simulink model "bmsfinal"  (R2026a)
settings: Solver=VariableStepAuto  StopTime=1000.0
libraries: fl_lib x3, nesl_utility x3, ee_lib x1, batteryecm_lib x1
settings Model: LastModifiedBy=amrut

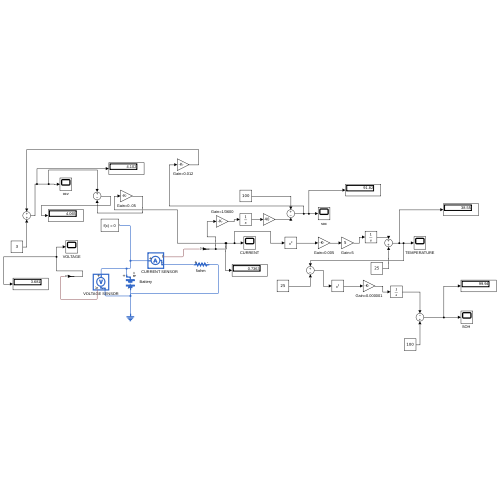
[thumbnail: Simulink's stored preview of the top-level diagram]
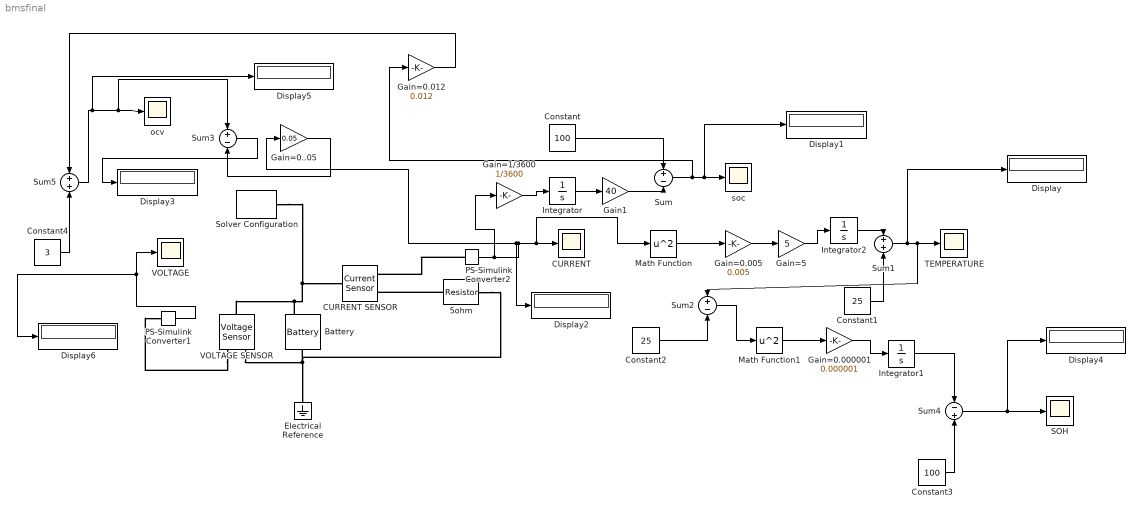
== system bmsfinal ==
  "          CURRENT SENSOR   " : fl_lib/Electrical/Electrical Sensors/Current Sensor
  5ohm : ee_lib/Passive/Resistor  R=5 Ohm  enable_R_tol=ee.enum.toleranceApplication.none  R_tol=5  tol_distribution=ee.enum.toleranceDistribution.uniform  nSigma=4  enable_operating_limits=ee.enum.enable.no  operating_limit_action=ee.enum.passive.reportOpLim.warn  power_rating=1 W  max_working_voltage=100 V  noise_mode=ee.enum.sources.noise.Disabled  Tdevice=25 degC  sample_time=1e-3 s  repeatability=ee.enum.ic.repeatability.notRepeatable  user_seed=0  auto_seed=3499211588  power_derating_T1=70 degC  power_derating_T2=155 degC  operating_temperature_range_vec=[-50, 150] degC  alpha=3.93e-3 1/K  Tmeas=25 degC  thermal_mass=100 J/K  temperature_specify=off  temperature_priority=High  temperature=298.15 K  temperature_nominal_specify=off  temperature_nominal_value=1  temperature_nominal_unit=K
  "Battery " : batteryecm_lib/Battery  Vnom=3.7 V  prm_dir=simscape.enum.battery.prm_dir.disabled  R1_dis=2 Ohm  R1_ch=2 Ohm  R1=0.05 Ohm  prm_AH=simscape.enum.battery.prm_AH.finite  AH=25 A*hr  V1=3.4 V  AH1=2.5 A*hr  prm_R2=simscape.enum.battery.prm_R2.disabled  R2=2000 Ohm  Tmeas=298.15 K  charge_measurement_port=simscape.enum.battery.enable.yes  prm_dyn=simscape.enum.battery.prm_dyn.off  Rp1=0.005 Ohm  tau1=30 s  Rp2=0.005 Ohm  tau2=30 s  Rp3=0.005 Ohm  tau3=30 s  Rp4=0.005 Ohm  tau4=30 s  Rp5=0.005 Ohm  tau5=30 s  prm_fade=simscape.enum.battery.prm_fade.disabled  N_fade=100  AH_fade=45 A*hr  R1_fade=2.02 Ohm  R1_ch_fade=2.02 Ohm  V1_fade=10.35 V  prm_age=simscape.enum.battery.prm_age.disabled  prm_age_OCV=simscape.enum.battery.prm_age_OCV.OCV  OCV_age=0.9  SOC_age=60  Tmeas_age=298.15 K  delta_time_age_vec=[0] d  temperature_age_vec=[273] K  OCV_scaling_age=2.2134e6  OCV_offset_age=1.632e6  temp_exp_age=0.515833569 V  t_exp_age=0.75  Vnom_T2=12 V  R1_T2=2.2 Ohm  R1_T2_dis=2.2 Ohm  R1_T2_ch=2.2 Ohm  V1_T2=11.4 V  R2_T2=2200 Ohm  Rp1_T2=0.005 Ohm  tau1_T2=30 s  Rp2_T2=0.005 Ohm  tau2_T2=30 s  Rp3_T2=0.005 Ohm  tau3_T2=30 s  Rp4_T2=0.005 Ohm  tau4_T2=30 s  Rp5_T2=0.005 Ohm  tau5_T2=30 s  Tmeas2=273.15 K  thermal_port=simscape.enum.thermaleffects.omit  thermal_mass=30000 J/K  i_specify=off  i_priority=None  i=0 A  i_nominal_specify=off  i_nominal_value=1  i_nominal_unit=A  v_specify=off  v_priority=None  v=0 V  v_nominal_specify=off  v_nominal_value=1  v_nominal_unit=V  charge_specify=off  charge_priority=High  charge=50 A*hr  charge_nominal_specify=off  charge_nominal_value=1  charge_nominal_unit=A*hr  num_cycles_specify=off  num_cycles_priority=High  num_cycles=0  num_cycles_nominal_specify=off  num_cycles_nominal_value=1  num_cycles_nominal_unit=1  temperature_specify=off  temperature_priority=High  temperature=298.15 K  temperature_nominal_specify=off  temperature_nominal_value=1  temperature_nominal_unit=K
  CURRENT : Scope
      settings: ActiveDisplayYMinimum=0.73628082550287643  ActiveDisplayYMaximum=0.73628268077145642
  Constant : Constant  Value=100
  Constant1 : Constant  Value=25
  Constant2 : Constant  Value=25
  Constant3 : Constant  Value=100
  Constant4 : Constant  Value=3
  Display{,1..6} (7 alike) : Display
  Electrical Reference : fl_lib/Electrical/Electrical Elements/Electrical Reference
  Gain1 : Gain  Gain=40
  Gain=0..05 : Gain  Gain=0.05
  Gain=0.000001 : Gain  Gain=0.000001
  Gain=0.005 : Gain  Gain=0.005
  Gain=0.012 : Gain  Gain=0.012
  Gain=1/3600 : Gain  Gain=1/3600
  Gain=5 : Gain  Gain=5
  Integrator : Integrator
  Integrator1 : Integrator
  Integrator2 : Integrator
  Math Function : Math  Operator=square
  Math Function1 : Math  Operator=square
  PS-Simulink Converter1 : nesl_utility/PS-Simulink Converter  PhysicalDomain=network_engine_domain  SubClassName=ps_output  LeftPortType=input  RightPortType=output  PseudoPeriodic=off  Frequencies=[]  VectorFormat=inherit  Unit=inherit  AffineConversion=off
  PS-Simulink Converter2 : nesl_utility/PS-Simulink Converter  PhysicalDomain=network_engine_domain  SubClassName=ps_output  LeftPortType=input  RightPortType=output  PseudoPeriodic=off  Frequencies=[]  VectorFormat=inherit  Unit=inherit  AffineConversion=off
  "SOH " : Scope
      settings: ActiveDisplayYMinimum=99.931095502685864  ActiveDisplayYMaximum=100.00765605525713  DataLoggingVariableName=ScopeData4
  Solver Configuration : nesl_utility/Solver Configuration  PhysicalDomain=network_engine_domain  SubClassName=solver  LeftPortType=input  RightPortType=generic  Tones=[]  Harmonics=[]  SimulateNoise=off  Profile=off  UseLocalSampling=off  EnableSwitchedLinearOptims=on  FrequencyDomain=off  UseCCode=off  RelTol=0.001  AbsTol=0.001  MinStep=1e-09  ToWorkspace=off  RevertToSquareIcSolve=off  NumHomotopyIterations=100  PhasorMode=off  PhasorModeNumHarmonics=1  ConsistencySolver=NEWTON_XTOL_AFTER_FTOL  CanonicalOrdering=CANONICAL  OptimizeIntermediates=OPTIMIZED  IndexReductionMethod=DerivativeReplacement  DoDC=off  ResidualTolerance=1e-09  ConsistencyTolSource=GLOBAL  ConsistencyAbsTol=0.001  ConsistencyRelTol=0.001  ConsistencyTolFactor=0.001  UseLocalSolver=off  LocalSolverChoice=NE_BACKWARD_EULER_ADVANCER  ResolveIndetEquations=on  FunctionEvalNumThread=1  LocalSolverSampleTime=0.001  DoFixedCost=off  MaxNonlinIter=3  MaxModeIter=2  ComputeImpulses=off  ImpulseIterations=2  LinearAlgebra=auto  LinearAlgebraNumThread=0  EquationFormulation=NE_TIME_EF  DelaysMemoryBudget=1024  AutomaticFiltering=on  FilteringTimeConstant=0.001  PartitionStorageMethod=AS_NEEDED  PartitionMemoryBudget=1024  PartitionMethod=ROBUST  MultibodyUseLocalSolver=off  MultibodyLocalSolverChoice=ODE1  MultibodyLocalSolverSampleTime=0.001
  Sum : Sum  Inputs=+-
  Sum1 : Sum
  Sum2 : Sum  Inputs=+-
  Sum3 : Sum  Inputs=+-
  Sum4 : Sum  Inputs=-+
  Sum5 : Sum
  TEMPERATURE : Scope
      settings: ActiveDisplayYMinimum=23.305934501032183  ActiveDisplayYMaximum=40.246589490710349  DataLoggingVariableName=ScopeData3
  VOLTAGE : Scope
      settings: ActiveDisplayYMinimum=3.6813286828160332  ActiveDisplayYMaximum=3.6814217866015433
  VOLTAGE SENSOR : fl_lib/Electrical/Electrical Sensors/Voltage Sensor
  ocv : Scope
      settings: ActiveDisplayYMinimum=4.089558741440749  ActiveDisplayYMaximum=4.2122712509510283  DataLoggingVariableName=ScopeData5
  soc : Scope
      settings: ActiveDisplayYMinimum=90.796561786729015  ActiveDisplayYMaximum=101.022604245919  DataLoggingVariableName=ScopeData2
  wires:
  PS-Simulink Converter1/1 -> Display6/1, VOLTAGE/1
  PS-Simulink Converter2/1 -> Gain=1/3600/1, Math Function/1, CURRENT/1, Gain=0..05/1, Display2/1
  Gain=1/3600/1 -> Integrator/1
  Integrator/1 -> Gain1/1
  Gain1/1 -> Sum/2
  Constant/1 -> Sum/1
  Sum/1 -> Gain=0.012/1, Display1/1, soc/1
  Math Function/1 -> Gain=0.005/1
  Gain=0.005/1 -> Gain=5/1
  Constant1/1 -> Sum1/2
  Sum1/1 -> Display/1, Sum2/1, TEMPERATURE/1
  Constant2/1 -> Sum2/2
  Sum2/1 -> Math Function1/1
  Math Function1/1 -> Gain=0.000001/1
  Gain=0.000001/1 -> Integrator1/1
  Integrator1/1 -> Sum4/1
  Constant3/1 -> Sum4/2
  Sum4/1 -> Display4/1, "SOH "/1
  Gain=0.012/1 -> Sum5/1
  Constant4/1 -> Sum5/2
  Sum5/1 -> Display5/1, Sum3/1, ocv/1
  Sum3/1 -> Display3/1
  Gain=0..05/1 -> Sum3/2
  Gain=5/1 -> Integrator2/1
  Integrator2/1 -> Sum1/1
  connections:
  "Battery "/LConn1 -- Solver Configuration/RConn1 -- "          CURRENT SENSOR   "/LConn1 -- VOLTAGE SENSOR/LConn1
  5ohm/LConn1 -- "          CURRENT SENSOR   "/RConn2
  5ohm/RConn1 -- VOLTAGE SENSOR/RConn2 -- Electrical Reference/LConn1 -- "Battery "/RConn1
  VOLTAGE SENSOR/RConn1 -- PS-Simulink Converter1/LConn1
  PS-Simulink Converter2/LConn1 -- "          CURRENT SENSOR   "/RConn1
